simulink model "Part2A"  (R2024a)
settings: Solver=VariableStepAuto  StartTime=0.0  StopTime=10.0  RelTol=1e-3
settings Model: Creator=kyleo  LastModifiedBy=kyleo

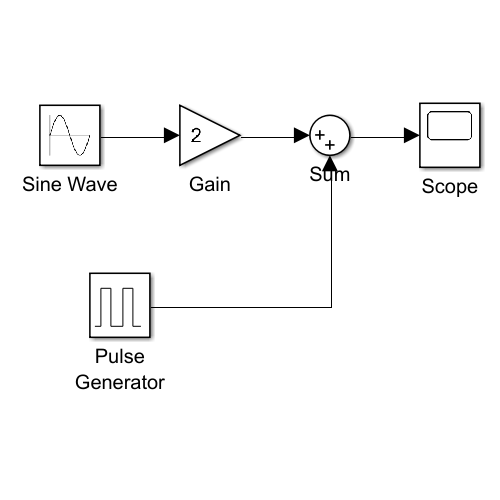
[thumbnail: Simulink's stored preview of the top-level diagram]
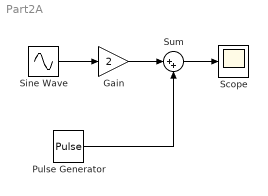
== system Part2A ==
  Gain : Gain  Gain=2
  Pulse Generator : DiscretePulseGenerator  PulseType=Time based  Amplitude=-1  Period=0.5  PulseWidth=50
  Scope : Scope
  Sine Wave : Sin  SampleTime=0
  Sum : Sum  Inputs=|++
  wires:
  Sum/1 -> Scope/1
  Sine Wave/1 -> Gain/1
  Gain/1 -> Sum/1
  Pulse Generator/1 -> Sum/2
